simulink model "version2A"  (R2021a)
settings: Solver=VariableStepAuto  StartTime=0.0  StopTime=10.0  RelTol=1e-3
undefined symbols (not defined in the file): J, P, Rs
settings Model: Creator=Aashish Kalra  LastModifiedBy=Aashish Kalra
settings OptimizationCC: DefaultUnderspecifiedDataType=single
settings DebuggingCC: UniqueDataStoreMsg=error  StrictBusMsg=ErrorOnBusTreatedAsVector

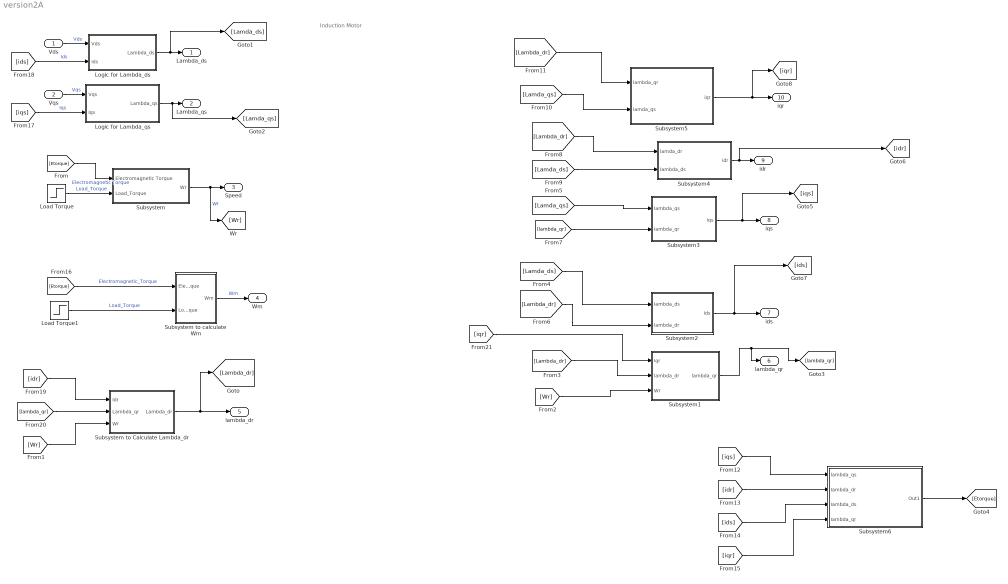
== system version2A ==
  note: Induction Motor
  Vds : Inport
  Vqs : Inport  Port=2
  Load Torque : Step  Time=5  After=20  SampleTime=0
  Load Torque1 : Step  Time=5  After=20  SampleTime=0
  Logic for Lambda_ds : Subsystem
  Logic for Lambda_qs : Subsystem
  Subsystem : Subsystem
  Subsystem to Calculate Lambda_dr : Subsystem
  Subsystem to calculate Wm : Subsystem
  Subsystem1 : Subsystem
  Subsystem2 : Subsystem
  Subsystem3 : Subsystem
  Subsystem4 : Subsystem
  Subsystem5 : Subsystem
  Subsystem6 : Subsystem
  Lambda_ds : Outport
  Lambda_qs : Outport  Port=2
  Speed : Outport  Port=3
  Wm : Outport  Port=4
  lambda_dr : Outport  Port=5
  lambda_qr : Outport  Port=6
  ids : Outport  Port=7
  iqs : Outport  Port=8
  idr : Outport  Port=9
  iqr : Outport  Port=10
  wires:
  Logic for Lambda_qs/1(Lambda_qs) -> [Lamda_qs], Lambda_qs/1
  Vds/1 -> Logic for Lambda_ds/1(Vds)  "Vds"
  [iqs] -> Logic for Lambda_qs/2(Iqs)  "Iqs"
  Vqs/1 -> Logic for Lambda_qs/1(Vqs)  "Vqs"
  Logic for Lambda_ds/1(Lambda_ds) -> [Lamda_ds], Lambda_ds/1
  [ids] -> Logic for Lambda_ds/2(Ids)  "Ids"
  [Etorque] -> Subsystem/1(Electromagnetic Torque)  "Electromagnetic Torque"
  Load Torque/1 -> Subsystem/2(Load_Torque)  "Load_Torque"
  Subsystem/1(Wr) -> [Wr], Speed/1  "Wr"
  [Etorque] -> Subsystem to calculate Wm/1(Electromagnetic_Torque)  "Electromagnetic_Torque"
  Load Torque1/1 -> Subsystem to calculate Wm/2(Load_Torque)  "Load_Torque"
  Subsystem to calculate Wm/1(Wm) -> Wm/1  "Wm"
  Subsystem to Calculate Lambda_dr/1(Lambda_dr) -> [Lambda_dr], lambda_dr/1
  [Wr] -> Subsystem to Calculate Lambda_dr/3(Wr)
  [iqr] -> Subsystem1/1(Iqr)
  [Wr] -> Subsystem1/3(Wr)
  Subsystem1/1(lambda_qr) -> [lambda_qr], lambda_qr/1
  [Lambda_dr] -> Subsystem1/2(lambda_dr)
  [Lamda_ds] -> Subsystem2/1(Iambda_ds)
  [Lambda_dr] -> Subsystem2/2(lambda_dr)
  Subsystem2/1(ids) -> [ids], ids/1
  [Lamda_qs] -> Subsystem3/1(Iambda_qs)
  [lambda_qr] -> Subsystem3/2(Iambda_qr)
  Subsystem3/1(iqs) -> [iqs], iqs/1
  [Lambda_dr] -> Subsystem4/1(lamda_dr)
  [Lamda_ds] -> Subsystem4/2(lambda_ds)
  Subsystem4/1(idr) -> [idr], idr/1
  [Lambda_dr] -> Subsystem5/1(lambda_qr)
  [Lamda_qs] -> Subsystem5/2(lamda_qs)
  Subsystem5/1(iqr) -> [iqr], iqr/1
  [iqs] -> Subsystem6/1(lambda_qs)
  [idr] -> Subsystem6/2(Iambda_dr)
  [ids] -> Subsystem6/3(Iambda_ds)
  [iqr] -> Subsystem6/4(Iambda_qr)
  Subsystem6/1(Out1) -> [Etorque]
  [idr] -> Subsystem to Calculate Lambda_dr/1(Idr)
  [lambda_qr] -> Subsystem to Calculate Lambda_dr/2(Lambda_qr)

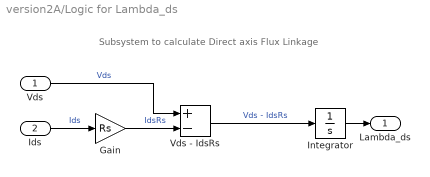
== system version2A/Logic for Lambda_ds ==
  note: Subsystem to calculate Direct axis Flux Linkage
  Vds : Inport
  Ids : Inport  Port=2
  Gain : Gain  Gain=Rs
  Integrator : Integrator
  Vds - IdsRs : Sum  Inputs=+-
  Lambda_ds : Outport
  wires:
  Ids/1 -> Gain/1  "Ids"
  Integrator/1 -> Lambda_ds/1
  Vds - IdsRs/1 -> Integrator/1  "Vds - IdsRs"
  Gain/1 -> Vds - IdsRs/2  "IdsRs"
  Vds/1 -> Vds - IdsRs/1  "Vds"

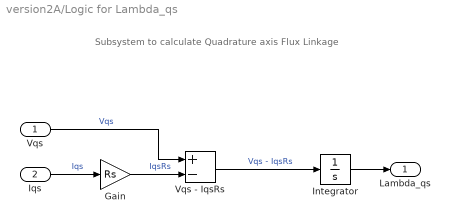
== system version2A/Logic for Lambda_qs ==
  note: Subsystem to calculate Quadrature axis Flux Linkage
  Vqs : Inport
  Iqs : Inport  Port=2
  Gain : Gain  Gain=Rs
  Integrator : Integrator
  Vqs - IqsRs : Sum  Inputs=+-
  Lambda_qs : Outport
  wires:
  Integrator/1 -> Lambda_qs/1
  Gain/1 -> Vqs - IqsRs/2  "IqsRs"
  Vqs - IqsRs/1 -> Integrator/1  "Vqs - IqsRs"
  Vqs/1 -> Vqs - IqsRs/1  "Vqs"
  Iqs/1 -> Gain/1  "Iqs"

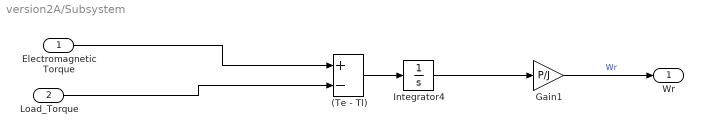
== system version2A/Subsystem ==
  Electromagnetic Torque : Inport
  Load_Torque : Inport  Port=2
  (Te - Tl) : Sum  Inputs=+-
  Gain1 : Gain  Gain=P/J
  Integrator4 : Integrator
  Wr : Outport
  wires:
  Load_Torque/1 -> (Te - Tl)/2
  Integrator4/1 -> Gain1/1
  (Te - Tl)/1 -> Integrator4/1
  Gain1/1 -> Wr/1  "Wr"
  Electromagnetic Torque/1 -> (Te - Tl)/1

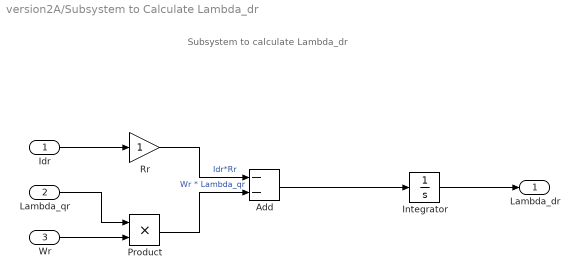
== system version2A/Subsystem to Calculate Lambda_dr ==
  note: Subsystem to calculate Lambda_dr
  Idr : Inport
  Lambda_qr : Inport  Port=2
  Wr : Inport  Port=3
  Add : Sum  Inputs=--
  Integrator : Integrator
  Product : Product
  Rr : Gain
  Lambda_dr : Outport
  wires:
  Add/1 -> Integrator/1
  Integrator/1 -> Lambda_dr/1
  Wr/1 -> Product/2
  Product/1 -> Add/2  "Wr * Lambda_qr"
  Lambda_qr/1 -> Product/1
  Idr/1 -> Rr/1
  Rr/1 -> Add/1  "Idr*Rr"

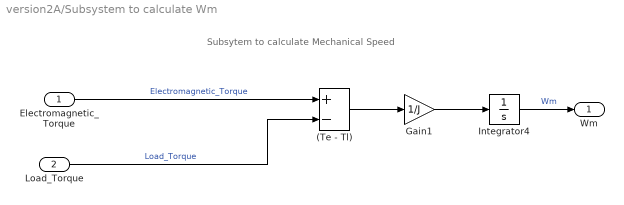
== system version2A/Subsystem to calculate Wm ==
  note: Subsytem to calculate Mechanical Speed
  Electromagnetic_Torque : Inport
  Load_Torque : Inport  Port=2
  (Te - Tl) : Sum  Inputs=+-
  Gain1 : Gain  Gain=1/J
  Integrator4 : Integrator
  Wm : Outport
  wires:
  Gain1/1 -> Integrator4/1
  Load_Torque/1 -> (Te - Tl)/2  "Load_Torque"
  Integrator4/1 -> Wm/1  "Wm"
  Electromagnetic_Torque/1 -> (Te - Tl)/1  "Electromagnetic_Torque"
  (Te - Tl)/1 -> Gain1/1

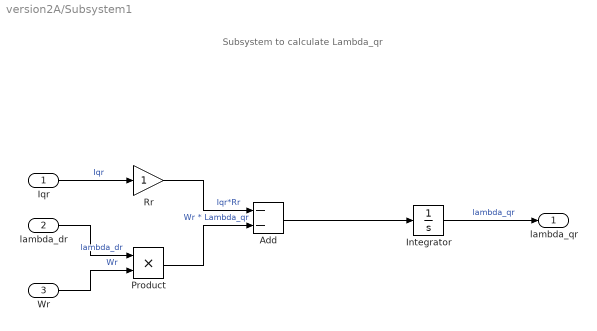
== system version2A/Subsystem1 ==
  note: Subsystem to calculate Lambda_qr
  Iqr : Inport
  lambda_dr : Inport  Port=2
  Wr : Inport  Port=3
  Add : Sum  Inputs=--
  Integrator : Integrator
  Product : Product
  Rr : Gain
  lambda_qr : Outport
  wires:
  Rr/1 -> Add/1  "Iqr*Rr"
  Product/1 -> Add/2  "Wr * Lambda_qr"
  Add/1 -> Integrator/1
  Integrator/1 -> lambda_qr/1  "lambda_qr"
  Iqr/1 -> Rr/1  "Iqr"
  Wr/1 -> Product/2  "Wr"
  lambda_dr/1 -> Product/1  "lambda_dr"

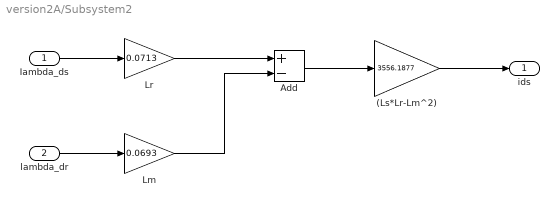
== system version2A/Subsystem2 ==
  Iambda_ds : Inport
  lambda_dr : Inport  Port=2
  (Ls*Lr-Lm^2) : Gain  Gain=3556.1877
  Add : Sum  Inputs=+-
  Lm : Gain  Gain=0.0693
  Lr : Gain  Gain=0.0713
  ids : Outport
  wires:
  (Ls*Lr-Lm^2)/1 -> ids/1
  Iambda_ds/1 -> Lr/1
  Lm/1 -> Add/2
  Add/1 -> (Ls*Lr-Lm^2)/1
  Lr/1 -> Add/1
  lambda_dr/1 -> Lm/1

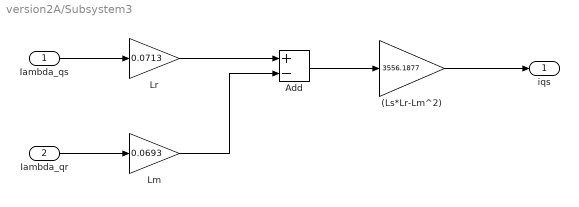
== system version2A/Subsystem3 ==
  Iambda_qs : Inport
  Iambda_qr : Inport  Port=2
  (Ls*Lr-Lm^2) : Gain  Gain=3556.1877
  Add : Sum  Inputs=+-
  Lm : Gain  Gain=0.0693
  Lr : Gain  Gain=0.0713
  iqs : Outport
  wires:
  Lr/1 -> Add/1
  Add/1 -> (Ls*Lr-Lm^2)/1
  (Ls*Lr-Lm^2)/1 -> iqs/1
  Lm/1 -> Add/2
  Iambda_qs/1 -> Lr/1
  Iambda_qr/1 -> Lm/1

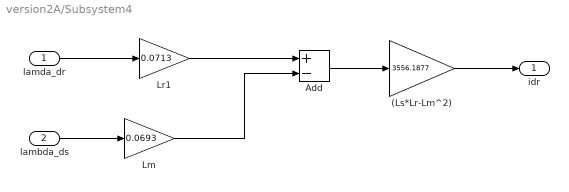
== system version2A/Subsystem4 ==
  lamda_dr : Inport
  lambda_ds : Inport  Port=2
  (Ls*Lr-Lm^2) : Gain  Gain=3556.1877
  Add : Sum  Inputs=+-
  Lm : Gain  Gain=0.0693
  Lr1 : Gain  Gain=0.0713
  idr : Outport
  wires:
  Lr1/1 -> Add/1
  Add/1 -> (Ls*Lr-Lm^2)/1
  (Ls*Lr-Lm^2)/1 -> idr/1
  lamda_dr/1 -> Lr1/1
  Lm/1 -> Add/2
  lambda_ds/1 -> Lm/1

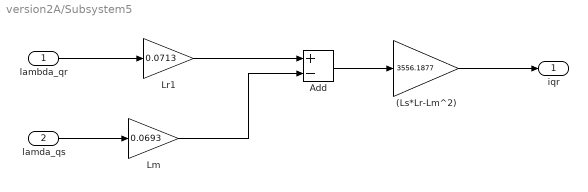
== system version2A/Subsystem5 ==
  lambda_qr : Inport
  lamda_qs : Inport  Port=2
  (Ls*Lr-Lm^2) : Gain  Gain=3556.1877
  Add : Sum  Inputs=+-
  Lm : Gain  Gain=0.0693
  Lr1 : Gain  Gain=0.0713
  iqr : Outport
  wires:
  Lm/1 -> Add/2
  Lr1/1 -> Add/1
  (Ls*Lr-Lm^2)/1 -> iqr/1
  Add/1 -> (Ls*Lr-Lm^2)/1
  lambda_qr/1 -> Lr1/1
  lamda_qs/1 -> Lm/1

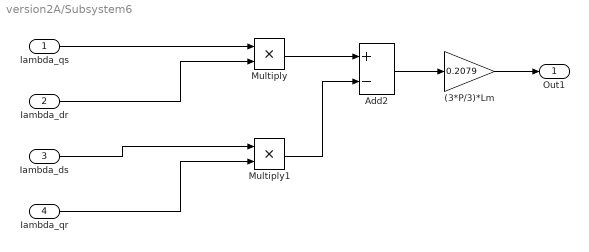
== system version2A/Subsystem6 ==
  lambda_qs : Inport
  Iambda_dr : Inport  Port=2
  Iambda_ds : Inport  Port=3
  Iambda_qr : Inport  Port=4
  (3*P/3)*Lm : Gain  Gain=0.2079
  Add2 : Sum  Inputs=+-
  Multiply : Product
  Multiply1 : Product
  Out1 : Outport
  wires:
  lambda_qs/1 -> Multiply/1
  Add2/1 -> (3*P/3)*Lm/1
  Multiply/1 -> Add2/1
  Iambda_qr/1 -> Multiply1/2
  Iambda_ds/1 -> Multiply1/1
  Multiply1/1 -> Add2/2
  (3*P/3)*Lm/1 -> Out1/1
  Iambda_dr/1 -> Multiply/2
